simulink model "PiSimulink_RPi"  (R2020b)
settings: Solver=FixedStepDiscrete  StartTime=0.0  StopTime=inf  FixedStep=0.01  RelTol=1e-3  EnableMultiTasking=on
libraries: embdlinuxlib x2, simulink x1, raspberrypiCommlib x1
settings Model: Creator=Audesse  LastModifiedBy=prasa
settings SolverCC: PositivePriorityOrder=on
settings DataIOCC: ReturnWorkspaceOutputs=off
settings OptimizationCC: DefaultUnderspecifiedDataType=single  EnhancedBackFolding=on  PassReuseOutputArgsAs=Individual arguments  MaxStackSize=64  OptimizeBlockOrder=speed  DifferentSizesBufferReuse=on  OptimizationCustomize=off  EfficientTunableParamExpr=on
settings DebuggingCC: ParameterTunabilityLossMsg=error
settings HardwareCC: ProdBitPerPointer=32  ProdBitPerSizeT=32  ProdBitPerPtrDiffT=32  ProdLargestAtomicInteger=Long  ProdLargestAtomicFloat=Double  ProdWordSize=32  ProdLongLongMode=on  ProdHWDeviceType=ARM Compatible->ARM Cortex
settings SFSimCC: MATLABDynamicMemAlloc=off  CustomCodeUndefinedFunction=UseInterfaceOnly
settings RTWCC: Description=Embedded Coder  SystemTargetFile=ert.tlc  HardwareBoard=Raspberry Pi  TLCOptions="-aInlineSetEventsForThisBaseRateFcn=TLC_FALSE -aSuppressMultiTaskScheduler=TLC_FALSE  -aRateBasedStepFcn=0"  TemplateMakefile=ert_default_tmf  GenerateReport=on  Toolchain=GNU GCC Raspberry Pi  BuildConfiguration=Faster Runs  IncludeHyperlinkInReport=on  LaunchReport=on  GenerateTraceInfo=on  GenerateTraceReport=on  GenerateTraceReportSl=on  GenerateTraceReportSf=on  GenerateTraceReportEml=on
settings CodeAppCC: ForceParamTrailComments=on  IgnoreCustomStorageClasses=off  OperatorAnnotations=on  SimulinkDataObjDesc=on  SFDataObjDesc=on  InsertBlockDesc=on
settings ERTTargetCC: MatFileLogging=on  SupportVariableSizeSignals=on

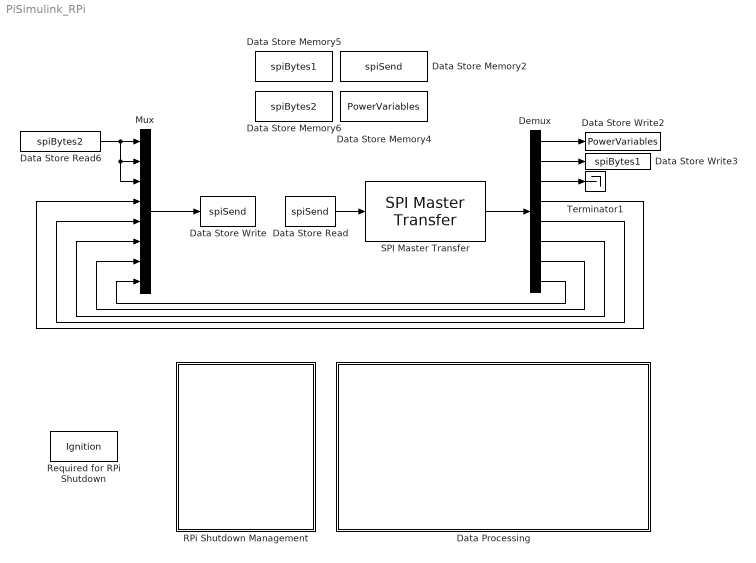
== system PiSimulink_RPi ==
  Data Processing : Subsystem
  Data Store Memory2 : DataStoreMemory  DataStoreName=spiSend  ReadBeforeWriteMsg=warning  WriteAfterWriteMsg=warning  WriteAfterReadMsg=warning  InitialValue=[0 0 0 0 0 0 0 0 0 0 0 0 0 0 0 0 0 0 0 0 0 0 0 0 0 0 0 0 0 0 0 0 0 0 0 0 0 0 0 0 0 0 0 0 0 0 0 0 0 0 0 0 0 0 0 0 0 0 0 0 0 0 0 0]  ShowAdditionalParam=off  OutDataTypeStr=uint8
  Data Store Memory4 : DataStoreMemory  DataStoreName=PowerVariables  ReadBeforeWriteMsg=warning  WriteAfterWriteMsg=warning  WriteAfterReadMsg=warning  InitialValue=[0 0 0 0 0 0 0 0]  ShowAdditionalParam=off  OutDataTypeStr=uint8
  Data Store Memory5 : DataStoreMemory  DataStoreName=spiBytes1  ReadBeforeWriteMsg=warning  WriteAfterWriteMsg=warning  WriteAfterReadMsg=warning  InitialValue=[255 255 255 255 255 255 255 255]  ShowAdditionalParam=off  OutDataTypeStr=uint8
  Data Store Memory6 : DataStoreMemory  DataStoreName=spiBytes2  ReadBeforeWriteMsg=warning  WriteAfterWriteMsg=warning  WriteAfterReadMsg=warning  InitialValue=[255 255 255 255 255 255 255 255]  ShowAdditionalParam=off  OutDataTypeStr=uint8
  Data Store Read : DataStoreRead  DataStoreName=spiSend
  Data Store Read6 : DataStoreRead  DataStoreName=spiBytes2
  Data Store Write : DataStoreWrite  DataStoreName=spiSend
  Data Store Write2 : DataStoreWrite  DataStoreName=PowerVariables
  Data Store Write3 : DataStoreWrite  DataStoreName=spiBytes1
  Demux : Demux  Outputs=8
  Mux : Mux  Inputs=8
  RPi Shutdown Management : Subsystem
  Required for RPi Shutdown : DataStoreMemory  DataStoreName=Ignition  ReadBeforeWriteMsg=warning  WriteAfterWriteMsg=warning  WriteAfterReadMsg=warning  ShowAdditionalParam=off  OutDataTypeStr=uint8
  SPI Master Transfer : raspberrypiCommlib/SPI Master Transfer  BoardProperty=Pi 4 Model B  SSPin=SPI0_CE0  SPIModule=uint32(0)  Mode=Master  BusSpeed=1000000  Pin=SPI0_CE0  FirstBitToTransfer=Most significant bit (MSB)  ClockMode=2  BlockFunction=Transfer  RegisterAddress=0  OutputDataType=int8  OutputDataLength=1
      settings: SourceProductBaseCode=RASPPI
  Terminator1 : Terminator
  wires:
  Data Store Read/1 -> SPI Master Transfer/1
  SPI Master Transfer/1 -> Demux/1
  Mux/1 -> Data Store Write/1
  Demux/2 -> Data Store Write3/1
  Demux/1 -> Data Store Write2/1
  Demux/7 -> Mux/7
  Demux/8 -> Mux/8
  Data Store Read6/1 -> Mux/3, Mux/2, Mux/1
  Demux/5 -> Mux/5
  Demux/4 -> Mux/4
  Demux/6 -> Mux/6
  Demux/3 -> Terminator1/1

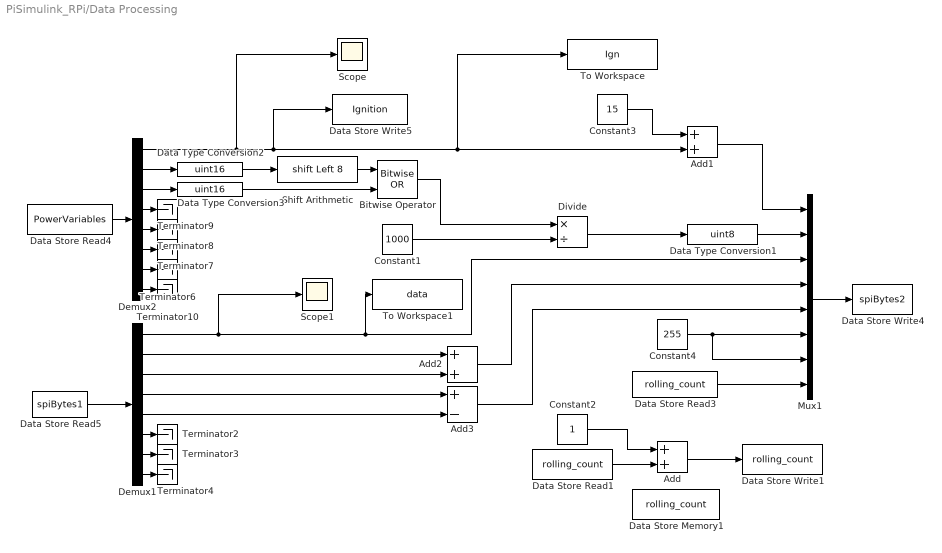
== system PiSimulink_RPi/Data Processing ==
  Add : Sum
  Add1 : Sum
  Add2 : Sum
  Add3 : Sum  Inputs=+-
  Bitwise Operator : simulink/Logic and Bit Operations/Bitwise Operator  logicop=OR  UseBitMask=off  NumInputPorts=2  BitMask=bin2dec('11011001')  BitMaskRealWorld=Stored Integer
  Constant1 : Constant  Value=1000  OutDataTypeStr=uint16
  Constant2 : Constant  OutDataTypeStr=uint8
  Constant3 : Constant  Value=15  OutDataTypeStr=uint8
  Constant4 : Constant  Value=255  OutDataTypeStr=uint8
  Data Store Memory1 : DataStoreMemory  DataStoreName=rolling_count  ReadBeforeWriteMsg=warning  WriteAfterWriteMsg=warning  WriteAfterReadMsg=warning  ShowAdditionalParam=off  OutDataTypeStr=uint8
  Data Store Read1 : DataStoreRead  DataStoreName=rolling_count
  Data Store Read3 : DataStoreRead  DataStoreName=rolling_count
  Data Store Read4 : DataStoreRead  DataStoreName=PowerVariables
  Data Store Read5 : DataStoreRead  DataStoreName=spiBytes1
  Data Store Write1 : DataStoreWrite  DataStoreName=rolling_count
  Data Store Write4 : DataStoreWrite  DataStoreName=spiBytes2
  Data Store Write5 : DataStoreWrite  DataStoreName=Ignition
  Data Type Conversion1 : DataTypeConversion  OutDataTypeStr=uint8
  Data Type Conversion2 : DataTypeConversion  OutDataTypeStr=uint16
  Data Type Conversion3 : DataTypeConversion  OutDataTypeStr=uint16
  Demux1 : Demux  Outputs=8
  Demux2 : Demux  Outputs=8
  Divide : Product  Inputs=*/  OutDataTypeStr=uint16
  Mux1 : Mux  Inputs=8
  Scope : Scope
  Scope1 : Scope
  Shift Arithmetic : ArithShift  BitShiftNumber=8  BitShiftDirection=Left
  Terminator{2..4,6..10} (8 alike) : Terminator
  To Workspace : ToWorkspace  VariableName=Ign  SampleTime=-1
      settings: Save2DSignal=2-D array (concatenate along first dimension)
  To Workspace1 : ToWorkspace  VariableName=data  SampleTime=-1
      settings: Save2DSignal=2-D array (concatenate along first dimension)
  wires:
  Constant4/1 -> Mux1/7, Mux1/6
  Constant2/1 -> Add/1
  Demux1/2 -> Add2/1
  Add/1 -> Data Store Write1/1
  Data Store Read1/1 -> Add/2
  Add1/1 -> Mux1/1
  Demux1/4 -> Add3/1
  Data Store Read5/1 -> Demux1/1
  Demux1/7 -> Terminator3/1
  Demux2/8 -> Terminator10/1
  Demux2/4 -> Terminator9/1
  Demux1/6 -> Terminator2/1
  Data Store Read4/1 -> Demux2/1
  Constant1/1 -> Divide/2
  Data Store Read3/1 -> Mux1/8
  Demux2/7 -> Terminator6/1
  Demux1/8 -> Terminator4/1
  Demux2/6 -> Terminator7/1
  Add2/1 -> Mux1/4
  Demux2/5 -> Terminator8/1
  Add3/1 -> Mux1/5
  Bitwise Operator/1 -> Divide/1
  Mux1/1 -> Data Store Write4/1
  Demux1/5 -> Add3/2
  Constant3/1 -> Add1/1
  Shift Arithmetic/1 -> Bitwise Operator/1
  Demux1/3 -> Add2/2
  Demux2/2 -> Data Type Conversion2/1
  Demux2/3 -> Data Type Conversion3/1
  Demux1/1 -> Scope1/1, To Workspace1/1, Mux1/3
  Data Type Conversion1/1 -> Mux1/2
  Divide/1 -> Data Type Conversion1/1
  Data Type Conversion2/1 -> Shift Arithmetic/1
  Data Type Conversion3/1 -> Bitwise Operator/2
  Demux2/1 -> Scope/1, To Workspace/1, Add1/2, Data Store Write5/1

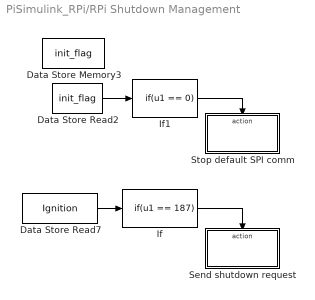
== system PiSimulink_RPi/RPi Shutdown Management ==
  Data Store Memory3 : DataStoreMemory  DataStoreName=init_flag  ReadBeforeWriteMsg=warning  WriteAfterWriteMsg=warning  WriteAfterReadMsg=warning  ShowAdditionalParam=off  OutDataTypeStr=uint8
  Data Store Read2 : DataStoreRead  DataStoreName=init_flag
  Data Store Read7 : DataStoreRead  DataStoreName=Ignition
  If : If  IfExpression=u1 == 187  ShowElse=off
  If1 : If  IfExpression=u1 == 0  ShowElse=off
  Send shutdown request : Subsystem  TreatAsAtomicUnit=on
  Stop default SPI comm : Subsystem  TreatAsAtomicUnit=on
  wires:
  If/1 -> Send shutdown request/Action
  Data Store Read7/1 -> If/1
  If1/1 -> Stop default SPI comm/Action
  Data Store Read2/1 -> If1/1

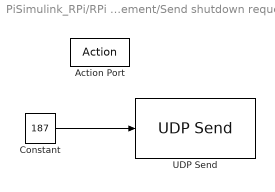
== system PiSimulink_RPi/RPi Shutdown Management/Send shutdown request ==
  Action Port : ActionPort  ActionPortLabel=if(u1 == 187)
  Constant : Constant  Value=187  OutDataTypeStr=uint8
  UDP Send : embdlinuxlib/UDP Send  remoteURL='127.0.0.1'  remotePort=5005  localURL='255.255.255.255'  localPortSource=Automatically determine  localPort=-1  sampletime=-1  blockPlatform=Raspberry Pi  separateLengthPort=0
      settings: SourceProductBaseCode=SC_BEAGLEBONE_BLUE,NVIDIA,RASPPI
  wires:
  Constant/1 -> UDP Send/1

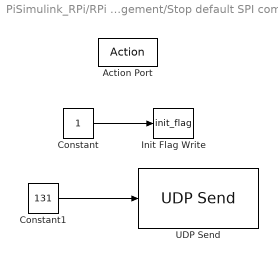
== system PiSimulink_RPi/RPi Shutdown Management/Stop default SPI comm ==
  Action Port : ActionPort  ActionPortLabel=if(u1 == 0)
  Constant : Constant  OutDataTypeStr=uint8
  Constant1 : Constant  Value=131  OutDataTypeStr=uint8
  Init Flag Write : DataStoreWrite  DataStoreName=init_flag
  UDP Send : embdlinuxlib/UDP Send  remoteURL='127.0.0.1'  remotePort=5005  localURL='255.255.255.255'  localPortSource=Automatically determine  localPort=-1  sampletime=-1  blockPlatform=Raspberry Pi  separateLengthPort=0
      settings: SourceProductBaseCode=SC_BEAGLEBONE_BLUE,NVIDIA,RASPPI
  wires:
  Constant/1 -> Init Flag Write/1
  Constant1/1 -> UDP Send/1
